simulink model "sampleModel1835"  (R2023a)
settings: Solver=VariableStepAuto  StartTime=0.0  StopTime=10.0  RelTol=1e-3
libraries: hdlsllib x6, simulink x1
settings Model: Creator=user1  LastModifiedBy=user1

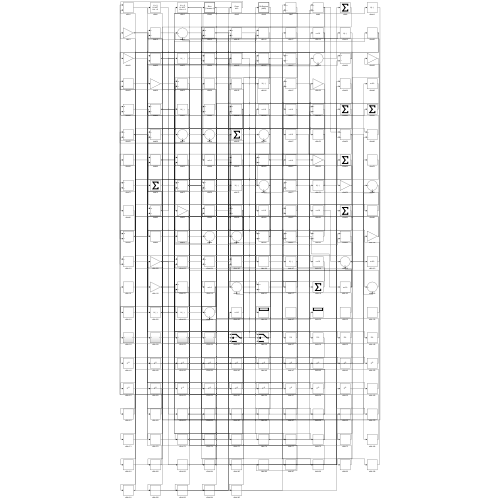
[thumbnail: Simulink's stored preview of the top-level diagram]
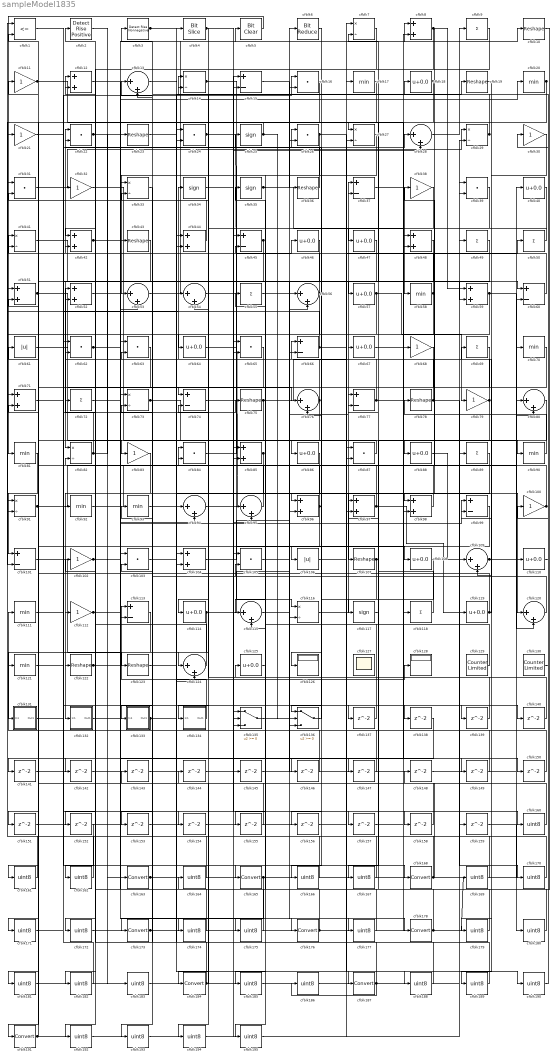
== system sampleModel1835 ==
  cfblk1 : RelationalOperator  Operator=<=  OutDataTypeStr=boolean  InputSameDT=off
  cfblk{10,19,23,36,43,75,78,107,122..123} (10 alike) : Reshape
  cfblk{11,21,30,32,38,68,79,83,100,102,112} (11 alike) : Gain
  cfblk{15,37,45,60,66,74,77,99,101,113} (10 alike) : Sum  Inputs=+-
  cfblk{16,22,24,26,31,39,62..63,65,84,87,103,105} (13 alike) : DotProduct  OutDataTypeStr=Inherit: Inherit via internal rule
  cfblk{8,12,42,44,48,51..52,59,71,85,96..98,104} (14 alike) : Sum
  cfblk106 : Abs  SaturateOnIntegerOverflow=off
  cfblk{18,40,46..47,57,64,67,86,88,108,110,114,119,125} (14 alike) : Bias  Bias=0.0  SaturateOnIntegerOverflow=off
  cfblk{13,28,53..54,56,76,80,94..95,109,115,120,124} (13 alike) : Sum  Inputs=|++
  cfblk{17,20,58,70,81,90,92..93,111,121} (10 alike) : MinMax
  cfblk{7,14,27,29,33,41,73,82,91,116} (10 alike) : Product  Inputs=*/  RndMeth=Zero  SaturateOnIntegerOverflow=on
  cfblk{25,34..35,117} (4 alike) : Signum
  cfblk{9,49..50,55,69,72,89,118} (8 alike) : Sum  Inputs=+
  cfblk126 : Display
  cfblk127 : Scope
      settings: Floating=on
  cfblk128 : Display
  cfblk129 : hdlsllib/Sources/Counter Limited  uplimit=7  tsamp=-1
  cfblk130 : hdlsllib/Sources/Counter Limited  uplimit=7  tsamp=-1
  cfblk131 : Subsystem
      settings: LibrarySourceBlock=|
      | hdlsllib/Ports &
      | Subsystems/Subsystem
  cfblk132 : Subsystem
      settings: LibrarySourceBlock=|
      | hdlsllib/Ports &
      | Subsystems/Subsystem
  cfblk133 : Subsystem
      settings: LibrarySourceBlock=|
      | hdlsllib/Ports &
      | Subsystems/Subsystem
  cfblk134 : Subsystem
      settings: LibrarySourceBlock=|
      | hdlsllib/Ports &
      | Subsystems/Subsystem
  cfblk135 : Switch  SaturateOnIntegerOverflow=off  InputSameDT=off
  cfblk136 : Switch  SaturateOnIntegerOverflow=off  InputSameDT=off
  cfblk{137..159} (23 alike) : Delay  SampleTime=1
  cfblk{160..162,164,166..167,169..172,174..175,177,179..183,185..186,188..190,192..195} (27 alike) : DataTypeConversion  OutDataTypeStr=uint8  SaturateOnIntegerOverflow=off  RndMeth=Floor
  cfblk{163,165,168,173,176,178,184,187,191} (9 alike) : DataTypeConversion  SaturateOnIntegerOverflow=off  RndMeth=Floor
  cfblk2 : hdlsllib/Logic and Bit Operations/Detect Rise Positive  vinit=0  OutDataTypeStr=boolean
  cfblk3 : hdlsllib/Logic and Bit Operations/Detect Rise Nonnegative  vinit=0  OutDataTypeStr=boolean
  cfblk4 : hdlsllib/Logic and Bit Operations/Bit Slice  lidx=7  ridx=0
  cfblk5 : simulink/Logic and Bit Operations/Bit Clear  iBit=0
      settings: LibrarySourceBlock=|
      | hdlsllib/Logic and Bit
      | Operations/Bit Clear
  cfblk6 : hdlsllib/Logic and Bit Operations/Bit Reduce  mode=AND
  cfblk61 : Abs  SaturateOnIntegerOverflow=off
  wires:
  cfblk14/1 -> cfblk106/1, cfblk28/2
  cfblk53/1 -> cfblk8/1
  cfblk87/1 -> cfblk86/1
  cfblk32/1 -> cfblk90/1
  cfblk64/1 -> cfblk116/1
  cfblk81/1 -> cfblk101/1
  cfblk134/1(Out1) -> cfblk113/1
  cfblk78/1 -> cfblk34/1, cfblk170/1
  cfblk110/1 -> cfblk18/1
  cfblk4/1 -> cfblk64/1, cfblk59/2
  cfblk38/1 -> cfblk124/1
  cfblk94/1 -> cfblk108/1
  cfblk24/1 -> cfblk95/1, cfblk158/1
  cfblk3/1 -> cfblk4/1, cfblk175/1
  cfblk41/1 -> cfblk60/1
  cfblk129/1 -> cfblk84/1
  cfblk51/1 -> cfblk83/1, cfblk138/1
  cfblk31/1 -> cfblk29/1
  cfblk48/1 -> cfblk82/1
  cfblk88/1 -> cfblk109/1
  cfblk5/1 -> cfblk81/1
  cfblk58/1 -> cfblk22/1, cfblk87/2, cfblk136/3
  cfblk25/1 -> cfblk21/1, cfblk136/2
  cfblk83/1 -> cfblk132/1(In1)
  cfblk116/1 -> cfblk37/1
  cfblk136/1 -> cfblk26/1
  cfblk90/1 -> cfblk78/1
  cfblk82/1 -> cfblk52/1, cfblk23/1
  cfblk37/1 -> cfblk58/1
  cfblk97/1 -> cfblk119/1, cfblk76/2
  cfblk66/1 -> cfblk126/1, cfblk50/1, cfblk14/1
  cfblk45/1 -> cfblk133/1(In1), cfblk114/1
  cfblk65/1 -> cfblk191/1
  cfblk72/1 -> cfblk176/1
  cfblk101/1 -> cfblk123/1
  cfblk57/1 -> cfblk79/1, cfblk174/1
  cfblk28/1 -> cfblk9/1
  cfblk112/1 -> cfblk25/1, cfblk99/1
  cfblk132/1(Out1) -> cfblk5/1
  cfblk122/1 -> cfblk10/1, cfblk84/2, cfblk192/1
  cfblk107/1 -> cfblk166/1, cfblk167/1
  cfblk74/1 -> cfblk107/1
  cfblk131/1(Out1) -> cfblk16/1
  cfblk91/1 -> cfblk80/1, cfblk54/1
  cfblk135/1 -> cfblk56/1
  cfblk27/1 -> cfblk53/1
  cfblk77/1 -> cfblk37/2, cfblk150/1
  cfblk102/1 -> cfblk135/2, cfblk177/1, cfblk183/1
  cfblk7/1 -> cfblk24/2
  cfblk133/1(Out1) -> cfblk111/1, cfblk128/1
  cfblk54/1 -> cfblk120/1
  cfblk86/1 -> cfblk96/1
  cfblk118/1 -> cfblk97/1
  cfblk52/1 -> cfblk73/1
  cfblk115/1 -> cfblk6/1
  cfblk85/1 -> cfblk112/1, cfblk104/2
  cfblk92/1 -> cfblk15/1
  cfblk99/1 -> cfblk122/1
  cfblk71/1 -> cfblk165/1
  cfblk95/1 -> cfblk41/1
  cfblk108/1 -> cfblk136/1
  cfblk36/1 -> cfblk12/1
  cfblk29/1 -> cfblk27/1, cfblk3/1
  cfblk84/1 -> cfblk46/1
  cfblk104/1 -> cfblk26/2
  cfblk121/1 -> cfblk28/1
  cfblk11/1 -> cfblk118/1, cfblk56/2
  cfblk61/1 -> cfblk105/1
  cfblk79/1 -> cfblk88/1, cfblk42/2
  cfblk22/1 -> cfblk139/1, cfblk140/1
  cfblk130/1 -> cfblk100/1
  cfblk8/1 -> cfblk98/1, cfblk59/1, cfblk44/2
  cfblk76/1 -> cfblk91/1, cfblk14/2
  cfblk70/1 -> cfblk74/1
  cfblk56/1 -> cfblk35/1, cfblk101/2
  cfblk35/1 -> cfblk98/2, cfblk185/1
  cfblk105/1 -> cfblk77/1
  cfblk100/1 -> cfblk38/1, cfblk74/2
  cfblk103/1 -> cfblk168/1
  cfblk60/1 -> cfblk11/1
  cfblk33/1 -> cfblk173/1
  cfblk119/1 -> cfblk31/2, cfblk13/1, cfblk99/2, cfblk54/2
  cfblk23/1 -> cfblk97/2
  cfblk16/1 -> cfblk91/2
  cfblk39/1 -> cfblk184/1
  cfblk125/1 -> cfblk45/2
  cfblk18/1 -> cfblk57/1, cfblk42/1
  cfblk98/1 -> cfblk51/2
  cfblk2/1 -> cfblk163/1
  cfblk20/1 -> cfblk109/2, cfblk181/1
  cfblk62/1 -> cfblk43/1, cfblk20/1
  cfblk109/1 -> cfblk70/1, cfblk120/2, cfblk69/1
  cfblk42/1 -> cfblk94/2, cfblk76/1, cfblk157/1
  cfblk44/1 -> cfblk12/2
  cfblk9/1 -> cfblk92/1
  cfblk55/1 -> cfblk178/1
  cfblk93/1 -> cfblk187/1
  cfblk67/1 -> cfblk48/2
  cfblk111/1 -> cfblk75/1
  cfblk50/1 -> cfblk47/1
  cfblk15/1 -> cfblk36/1
  cfblk26/1 -> cfblk190/1, cfblk195/1
  cfblk73/1 -> cfblk19/1, cfblk116/2, cfblk124/2, cfblk135/3
  cfblk124/1 -> cfblk102/1
  cfblk59/1 -> cfblk110/1, cfblk66/2
  cfblk96/1 -> cfblk66/1, cfblk63/2, cfblk141/1
  cfblk114/1 -> cfblk96/2, cfblk152/1, cfblk153/1
  cfblk75/1 -> cfblk134/1(In1), cfblk17/1
  cfblk120/1 -> cfblk105/2
  cfblk69/1 -> cfblk85/2
  cfblk113/1 -> cfblk131/1(In1)
  cfblk46/1 -> cfblk115/1
  cfblk43/1 -> cfblk121/1
  cfblk80/1 -> cfblk117/1
  cfblk117/1 -> cfblk77/2
  cfblk123/1 -> cfblk137/1
  cfblk137/1 -> cfblk51/1
  cfblk139/1 -> cfblk31/1
  cfblk140/1 -> cfblk52/2
  cfblk141/1 -> cfblk60/2
  cfblk47/1 -> cfblk142/1
  cfblk142/1 -> cfblk8/2
  cfblk143/1 -> cfblk95/2
  cfblk144/1 -> cfblk80/2
  cfblk145/1 -> cfblk16/2
  cfblk12/1 -> cfblk146/1
  cfblk146/1 -> cfblk24/1
  cfblk34/1 -> cfblk147/1
  cfblk147/1 -> cfblk45/1
  cfblk148/1 -> cfblk29/2
  cfblk13/1 -> cfblk149/1
  cfblk149/1 -> cfblk113/2
  cfblk150/1 -> cfblk82/2
  cfblk17/1 -> cfblk151/1
  cfblk151/1 -> cfblk53/2
  cfblk153/1 -> cfblk27/2
  cfblk21/1 -> cfblk154/1
  cfblk154/1 -> cfblk85/1
  cfblk40/1 -> cfblk155/1
  cfblk155/1 -> cfblk41/2
  cfblk6/1 -> cfblk156/1
  cfblk156/1 -> cfblk7/1
  cfblk157/1 -> cfblk48/1
  cfblk158/1 -> cfblk73/2
  cfblk1/1 -> cfblk160/1
  cfblk160/1 -> cfblk67/1
  cfblk138/1 -> cfblk161/1
  cfblk161/1 -> cfblk1/1
  cfblk152/1 -> cfblk162/1
  cfblk162/1 -> cfblk1/2
  cfblk163/1 -> cfblk44/1, cfblk40/1
  cfblk10/1 -> cfblk164/1
  cfblk164/1 -> cfblk2/1
  cfblk165/1 -> cfblk125/1, cfblk193/1
  cfblk166/1 -> cfblk71/1
  cfblk167/1 -> cfblk71/2
  cfblk168/1 -> cfblk148/1, cfblk13/2
  cfblk169/1 -> cfblk103/1
  cfblk170/1 -> cfblk103/2
  cfblk68/1 -> cfblk171/1
  cfblk171/1 -> cfblk32/1
  cfblk63/1 -> cfblk172/1
  cfblk172/1 -> cfblk68/1
  cfblk173/1 -> cfblk94/1, cfblk15/2
  cfblk174/1 -> cfblk33/1
  cfblk175/1 -> cfblk33/2
  cfblk176/1 -> cfblk169/1, cfblk63/1
  cfblk177/1 -> cfblk72/1
  cfblk178/1 -> cfblk115/2, cfblk7/2
  cfblk19/1 -> cfblk179/1
  cfblk179/1 -> cfblk55/1
  cfblk159/1 -> cfblk180/1
  cfblk180/1 -> cfblk62/2
  cfblk181/1 -> cfblk159/1
  cfblk89/1 -> cfblk182/1
  cfblk182/1 -> cfblk62/1
  cfblk183/1 -> cfblk89/1
  cfblk184/1 -> cfblk144/1, cfblk104/1
  cfblk185/1 -> cfblk39/1
  cfblk186/1 -> cfblk39/2
  cfblk187/1 -> cfblk186/1, cfblk143/1, cfblk135/1
  cfblk106/1 -> cfblk188/1
  cfblk188/1 -> cfblk93/1
  cfblk30/1 -> cfblk189/1
  cfblk189/1 -> cfblk22/2
  cfblk190/1 -> cfblk30/1
  cfblk191/1 -> cfblk61/1, cfblk87/1
  cfblk192/1 -> cfblk65/1
  cfblk193/1 -> cfblk65/2
  cfblk49/1 -> cfblk194/1
  cfblk194/1 -> cfblk145/1
  cfblk195/1 -> cfblk49/1

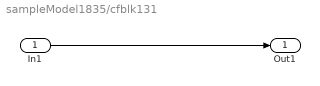
== system sampleModel1835/cfblk131 ==
  In1 : Inport
  Out1 : Outport
  wires:
  In1/1 -> Out1/1

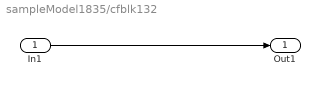
== system sampleModel1835/cfblk132 ==
  In1 : Inport
  Out1 : Outport
  wires:
  In1/1 -> Out1/1

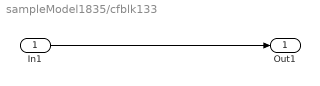
== system sampleModel1835/cfblk133 ==
  In1 : Inport
  Out1 : Outport
  wires:
  In1/1 -> Out1/1

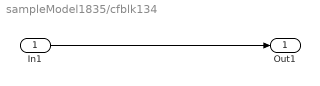
== system sampleModel1835/cfblk134 ==
  In1 : Inport
  Out1 : Outport
  wires:
  In1/1 -> Out1/1
